simulink model "tire_forces_fl_fr"  (R2015a)
settings: Solver=ode45  StartTime=0.0  StopTime=10.0  RelTol=1e-3
settings Model: Creator=BML  LastModifiedBy=BML

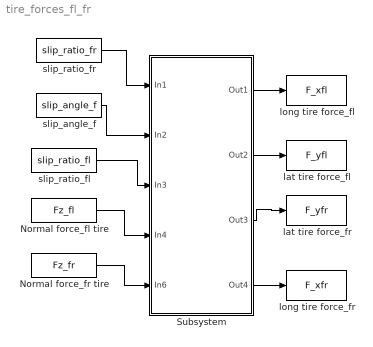
== system tire_forces_fl_fr ==
  Normal force_fl tire : FromWorkspace  VariableName=Fz_fl  SampleTime=0
  Normal force_fr tire : FromWorkspace  VariableName=Fz_fr  SampleTime=0
  Subsystem : Subsystem
  lat tire force_fl : ToWorkspace  VariableName=F_yfl  SaveFormat=Timeseries  SampleTime=-1
  lat tire force_fr : ToWorkspace  VariableName=F_yfr  SaveFormat=Timeseries  SampleTime=-1
  long tire force_fl : ToWorkspace  VariableName=F_xfl  SaveFormat=Timeseries  SampleTime=-1
  long tire force_fr : ToWorkspace  VariableName=F_xfr  SaveFormat=Timeseries  SampleTime=-1
  slip_angle_f : FromWorkspace  VariableName=slip_angle_f  SampleTime=0
  slip_ratio_fl : FromWorkspace  VariableName=slip_ratio_fl  SampleTime=0
  slip_ratio_fr : FromWorkspace  VariableName=slip_ratio_fr  SampleTime=0
  wires:
  slip_ratio_fr/1 -> Subsystem/1(In1)
  slip_angle_f/1 -> Subsystem/2(In2)
  slip_ratio_fl/1 -> Subsystem/3(In3)
  Normal force_fl tire/1 -> Subsystem/4(In4)
  Normal force_fr tire/1 -> Subsystem/5(In6)
  Subsystem/1(Out1) -> long tire force_fl/1
  Subsystem/2(Out2) -> lat tire force_fl/1
  Subsystem/3(Out3) -> lat tire force_fr/1
  Subsystem/4(Out4) -> long tire force_fr/1

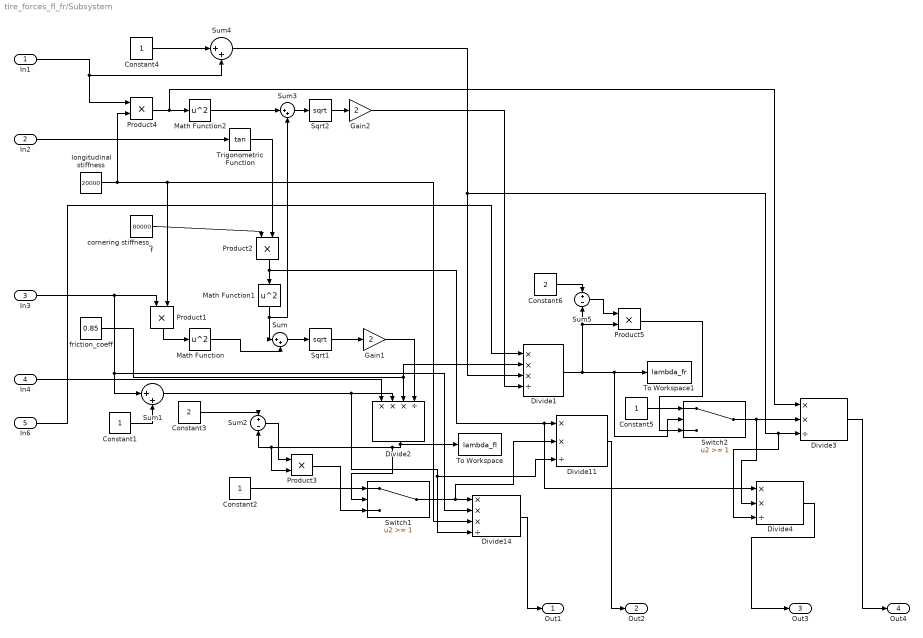
== system tire_forces_fl_fr/Subsystem ==
  In1 : Inport
  In2 : Inport  Port=2
  In3 : Inport  Port=3
  In4 : Inport  Port=4
  In6 : Inport  Port=5
  Constant{1..2,4..5} (4 alike) : Constant
  Constant3 : Constant  Value=2
  Constant6 : Constant  Value=2
  Divide1 : Product  Inputs=***/
  Divide11 : Product  Inputs=**/
  Divide14 : Product  Inputs=***/
  Divide2 : Product  Inputs=***/
  Divide3 : Product  Inputs=**/
  Divide4 : Product  Inputs=**/
  Gain1 : Gain  Gain=2
  Gain2 : Gain  Gain=2
  Math Function : Math  Operator=square  SaturateOnIntegerOverflow=on
  Math Function1 : Math  Operator=square  SaturateOnIntegerOverflow=on
  Math Function2 : Math  Operator=square  SaturateOnIntegerOverflow=on
  Product{1..5} (5 alike) : Product
  Sqrt1 : Sqrt  SaturateOnIntegerOverflow=on
  Sqrt2 : Sqrt  SaturateOnIntegerOverflow=on
  Sum{,1,3..4} (4 alike) : Sum  Inputs=|++
  Sum2 : Sum  Inputs=+-
  Sum5 : Sum  Inputs=+-
  Switch1 : Switch  Threshold=1
  Switch2 : Switch  Threshold=1
  To Workspace : ToWorkspace  VariableName=lambda_fl  SaveFormat=Timeseries  SampleTime=-1
  To Workspace1 : ToWorkspace  VariableName=lambda_fr  SaveFormat=Timeseries  SampleTime=-1
  Trigonometric Function : Trigonometry  Operator=tan
  cornering stiffness_f : Constant  Value=80000
  friction_coeff : Constant  Value=0.85
  longitudinal stiffness : Constant  Value=20000
  Out1 : Outport
  Out2 : Outport  Port=2
  Out3 : Outport  Port=3
  Out4 : Outport  Port=4
  wires:
  Math Function/1 -> Sum/2
  Constant1/1 -> Sum1/2
  Gain1/1 -> Divide2/4
  Trigonometric Function/1 -> Product2/2
  In3/1 -> Divide14/2, Sum1/1, Product1/1
  Sum/1 -> Sqrt1/1
  friction_coeff/1 -> Divide1/2, Divide2/3
  Sqrt1/1 -> Gain1/1
  In4/1 -> Divide2/1
  Product3/1 -> Switch1/3
  Gain2/1 -> Divide1/4
  Math Function1/1 -> Sum3/2, Sum/1
  Sum5/1 -> Product5/1
  Product2/1 -> Divide4/1, Divide11/1, Math Function1/1
  Constant5/1 -> Switch2/1
  cornering stiffness_f/1 -> Product2/1
  Switch2/1 -> Divide4/2, Divide3/2
  Divide14/1 -> Out1/1
  In6/1 -> Divide1/1
  Sum4/1 -> Divide4/3, Divide3/3, Divide1/3
  Constant2/1 -> Switch1/1
  Sum1/1 -> Divide11/3, Divide14/4, Divide2/2
  Divide11/1 -> Out2/1
  In1/1 -> Sum4/2, Product4/1
  Switch1/1 -> Divide11/2, Divide14/1
  Constant4/1 -> Sum4/1
  longitudinal stiffness/1 -> Product4/2, Product1/2, Divide14/3
  Sum3/1 -> Sqrt2/1
  Math Function2/1 -> Sum3/1
  Constant6/1 -> Sum5/1
  Sqrt2/1 -> Gain2/1
  Product4/1 -> Divide3/1, Math Function2/1
  Divide3/1 -> Out4/1
  Divide4/1 -> Out3/1
  Sum2/1 -> Product3/1
  Divide1/1 -> Switch2/2, To Workspace1/1, Sum5/2, Product5/2
  Constant3/1 -> Sum2/1
  Product1/1 -> Math Function/1
  In2/1 -> Trigonometric Function/1
  Divide2/1 -> Switch1/2, Product3/2, Sum2/2, To Workspace/1
  Product5/1 -> Switch2/3
